simulink model "xpcserialbinarytest_peter"  (Simulink 7.1)
settings: Solver=FixedStepDiscrete  StartTime=0.0  StopTime=inf  RelTol=1e-3
InitFcn:
  | trun = .1;
libraries: xpclib x4, simulink x2
Description:
  | Serial Blocks Loopback Test Using Binary Encoding/Decoding
  | 
  | This model demonstrates the BINARY FIFO read block in a form that can be simulated without using any specific serial hardware.  The input to the FIFO write block is the concatenation of several pieces comprising two separate 'messages'.  The first message is the byte stream: [170, 1, N] and the second is [170 2 44 M] where N is an incrementing number and M is a decrementing number.  The initial '8' in the first constant is the number of elements that follow.  The '5' is an extraneous value that shows how the FIFO binary read will ignore extra information.
  | 
  | To run this test with real serial port hardware, replace the FIFO write block with the send/receive block with FIFO OUT that corresponds to your hardware from the xpclib rs232 section. Then feed the output signal back to the input with a wire to perform a loopback test.
settings Model: Creator=gweast  LastModifiedBy=Administrator  ExtModeArmWhenConnect=off  BufferReuse=off
settings OptimizationCC: BlockReduction=off  OptimizeBlockIOStorage=off  BufferReuse=off  ExpressionFolding=off  FoldNonRolledExpr=off  LocalBlockOutputs=off
settings DebuggingCC: SaveWithParameterizedLinksMsg=none  SignalResolutionControl=TryResolveAllWithWarning  MultiTaskDSMMsg=warning  MultiTaskCondExecSysMsg=none  StrictBusMsg=None
settings HardwareCC: ProdIntDivRoundTo=Zero  ProdEndianess=LittleEndian  ProdHWDeviceType=Generic->32-bit x86 compatible
settings RTWCC: SystemTargetFile=xpctarget.tlc  TemplateMakefile=xpc_default_tmf  Description=xPC Target  ProcessScript=xpctarget_make_rtw_hook  IncludeERTFirstTime=on
settings xpcTargetCC: TargetFcnLib=ansi_tfl_tmw.mat  TargetFunctionLibrary=ANSI_C  CompOptLevelCompliant=off  PortableWordSizes=off  xPCisDownloadable=off

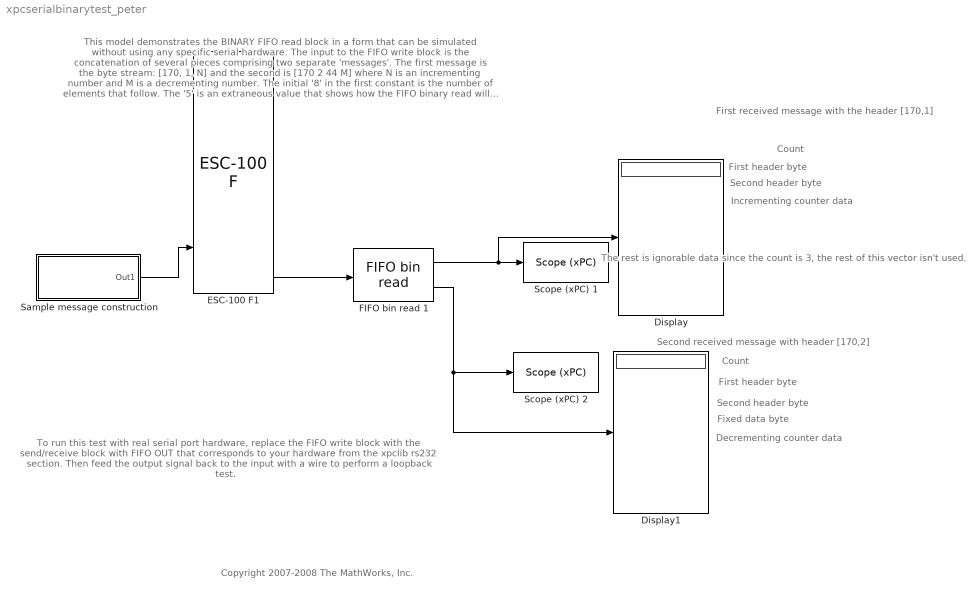
== system xpcserialbinarytest_peter ==
  note: This model demonstrates the BINARY FIFO read block in a form that can
      | be simulated without using any specific serial hardware.  The input to
      | the FIFO write block is the concatenation of several pieces comprising
      | two separate 'messages'.  The first message is the byte stream:
      | [170, 1, N] and the second is [170 2 44 M] where N is an incrementing
      | number and M is a decrementing number.  The initial '8' in the first constant
      | is the number of elements that follow.  The '5' is an extraneous value that
      | shows how the FIFO binary read will ignore extra information.
  note: To run this test with
      | real serial port hardware,
      | replace the FIFO write
      | block with the send/receive
      | block with FIFO OUT that
      | corresponds to your
      | hardware from the xpclib
      | rs232 section. Then feed
      | the output signal back to
      | the input with a wire to
      | perform a loopback test.
  note: First received message
      | with the header [170,1]
  note: Count
  note: First header byte
  note: Second header byte
  note: Incrementing counter data
  note: The rest is ignorable
      | data since the count
      | is 3, the rest of this
      | vector isn't used.
  note: Count
  note: First header byte
  note: Second header byte
  note: Fixed data byte
  note: Decrementing counter data
  note: Second received message
      | with header [170,2]
  note: Copyright 2007-2008 The MathWorks, Inc.
  Display : Display
  Display1 : Display
  ESC-100 F1 : xpclib/RS232/Quatech/ESC-100/ESC-100 F  SystemSampleTime=-1  group=FIFO Setup  port=8  irqnum=10  slot=-1  baud1=57600  parity1=None  ndata1=8  nstop1=1  fifomode1=64 deep  rlevel1=half full  automode1=off  xmtfifosize1=1024  xmtdatatype1=count+16 bit int  rcvfifosize1=1024  baud2=57600  parity2=None  ndata2=8  nstop2=1  fifomode2=64 deep  rlevel2=half full  automode2=off  xmtfifosize2=1024  xmtdatatype2=count+16 bit int  rcvfifosize2=1024  baud3=57600  parity3=None  ndata3=8  nstop3=1  fifomode3=64 deep  rlevel3=half full  automode3=off  xmtfifosize3=1024  xmtdatatype3=count+16 bit int  rcvfifosize3=1024  buad4=57600  parity4=None  ndata4=8  nstop4=1  fifomode4=64 deep  rlevel4=half full  automode4=off  xmtfifosize4=1024  xmtdatatype4=count+16 bit int  rcvfifosize4=1024  baud5=57600  parity5=None  ndata5=8  nstop5=1  fifomode5=64 deep  rlevel5=half full  automode5=off  xmtfifosize5=1024  xmtdatatype5=count+16 bit int  rcvfifosize5=1024  baud6=57600  parity6=None  ndata6=8  nstop6=1  fifomode6=64 deep  rlevel6=half full  automode6=off  xmtfifosize6=1024  xmtdatatype6=count+16 bit int  rcvfifosize6=1024  baud7=57600  parity7=None  ndata7=8  nstop7=1  fifomode7=64 deep  rlevel7=half full  automode7=off  xmtfifosize7=1024  xmtdatatype7=count+16 bit int  rcvfifosize7=1024  baud8=57600  parity8=None  ndata8=8  nstop8=1  fifomode8=64 deep  rlevel8=half full  automode8=off  xmtfifosize8=1024  xmtdatatype8=count+16 bit int  rcvfifosize8=1024
  FIFO bin read 1 : xpclib/RS232/FIFO bin read   header={char([170, 1]), char([170,2])}  lengths=[3 4]  hold=Zero output if no new data  enable=off  maxsize=6  outputtype=count+16 bit int  sampletime=trun
  Sample message construction : Subsystem
  Scope (xPC) 1 : xpclib/Misc./Scope (xPC)   SystemSampleTime=-1  scopeno=2  scopetype=Target  autostart=on  viewmode=Graphical sliding  formatstr='%15.6f'  grid=on  ylimits=[0,0]  nosamples=512  noprepostsamples=0  interleave=1  triggermode=FreeRun  triggersignal=1  triggerlevel=0.0  triggerslope=Either  triggerscope=1  triggersample=0  filename=data.dat  mode=Lazy  writesize=512  autorestart=off
  Scope (xPC) 2 : xpclib/Misc./Scope (xPC)   SystemSampleTime=-1  scopeno=1  scopetype=Target  autostart=on  viewmode=Graphical sliding  formatstr='%15.6f'  grid=on  ylimits=[0,0]  nosamples=512  noprepostsamples=0  interleave=1  triggermode=FreeRun  triggersignal=1  triggerlevel=0.0  triggerslope=Either  triggerscope=1  triggersample=0  filename=data.dat  mode=Lazy  writesize=512  autorestart=off
  wires:
  ESC-100 F1/8 -> FIFO bin read 1/1
  FIFO bin read 1/1 -> Scope (xPC) 1/1, Display/1
  FIFO bin read 1/2 -> Scope (xPC) 2/1, Display1/1
  Sample message construction/1(Out1) -> ESC-100 F1/7

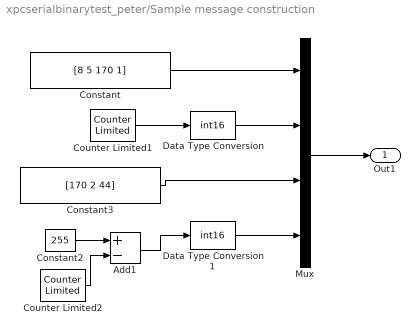
== system xpcserialbinarytest_peter/Sample message construction ==
  Add1 : Sum  Inputs=+-  OutDataType=sfix(16)  OutScaling=2^-10
  Constant : Constant  Value=[8 5 170 1]  OutDataTypeMode=int16  OutDataType=sfix(16)  OutScaling=2^0  OutDataTypeStr=int16
  Constant2 : Constant  Value=255  OutDataType=sfix(16)  OutScaling=2^0
  Constant3 : Constant  Value=[170 2 44]  OutDataTypeMode=int16  OutDataType=sfix(16)  OutScaling=2^0  OutDataTypeStr=int16
  Counter Limited1 : simulink/Sources/Counter Limited  SystemSampleTime=-1  uplimit=255  tsamp=trun
  Counter Limited2 : simulink/Sources/Counter Limited  SystemSampleTime=-1  uplimit=255  tsamp=trun
  Data Type Conversion : DataTypeConversion  OutDataTypeMode=int16  OutDataType=sfix(16)  OutScaling=2^0  OutDataTypeStr=int16
  Data Type Conversion1 : DataTypeConversion  OutDataTypeMode=int16  OutDataType=sfix(16)  OutScaling=2^0  OutDataTypeStr=int16
  Mux : Mux
  Out1 : Outport  OutDataType=sfix(16)  OutScaling=2^0
  wires:
  Counter Limited1/1 -> Data Type Conversion/1
  Constant/1 -> Mux/1
  Constant3/1 -> Mux/3
  Data Type Conversion/1 -> Mux/2
  Data Type Conversion1/1 -> Mux/4
  Mux/1 -> Out1/1
  Constant2/1 -> Add1/1
  Counter Limited2/1 -> Add1/2
  Add1/1 -> Data Type Conversion1/1
